simulink subsystem "transrapid_prebouclage"  (R2023a)
settings: Solver=VariableStepAuto  StartTime=0.0  StopTime=10.0  RelTol=1e-3
undefined symbols (not defined in the file): i0, k1, k2, kd, Ki, kp, Kz, Te, z0
libraries: dspsrcs4 x1
settings Model: Creator=leolebuhotel  LastModifiedBy=leolebuhotel

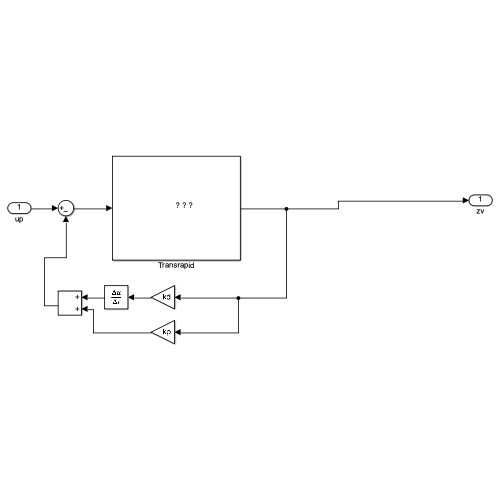
[thumbnail: Simulink's stored preview of the top-level diagram]
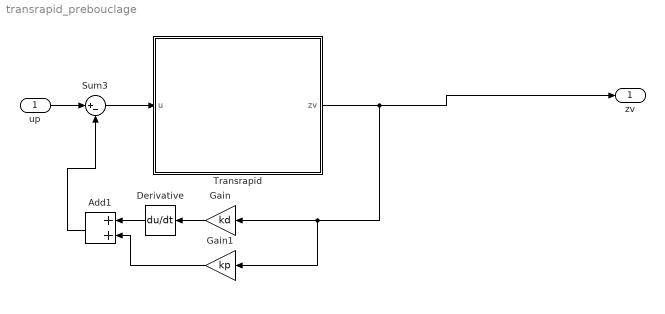
== system transrapid_prebouclage ==
  up : Inport
  Add1 : Sum
  Derivative : Derivative
  Gain : Gain  Gain=kd
  Gain1 : Gain  Gain=kp
  Sum3 : Sum  Inputs=|+-
  Transrapid : Subsystem
      mask Display:
      | image('Transrapid.jpg');
      | color('yellow')
      | port_label('output', 1, 'z');
      | port_label('input', 1, 'commande u');
  zv : Outport
  wires:
  Gain1/1 -> Add1/2
  Derivative/1 -> Add1/1
  up/1 -> Sum3/1
  Add1/1 -> Sum3/2
  Sum3/1 -> Transrapid/1(u)
  Transrapid/1(zv) -> zv/1, Gain1/1, Gain/1
  Gain/1 -> Derivative/1

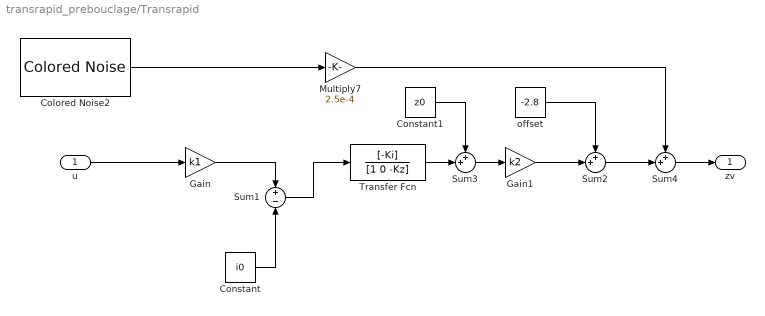
== system transrapid_prebouclage/Transrapid ==
  u : Inport
  Colored Noise2 : dspsrcs4/Colored Noise  Color=white  InverseFrequencyPower=1  BoundedOutput=off  NumChannels=1  OutputDataType=double  SamplesPerFrame=1  SampleTime=Te  RandomStream=mt19937ar with seed  Seed=67  SimulateUsing=Interpreted execution
  Constant : Constant  Value=i0
  Constant1 : Constant  Value=z0
  Gain : Gain  Gain=k1
  Gain1 : Gain  Gain=k2
  Multiply7 : Gain  Gain=2.5e-4
  Sum1 : Sum  Inputs=+-
  Sum2 : Sum  Inputs=++|
  Sum3 : Sum  Inputs=++|
  Sum4 : Sum  Inputs=++|
  Transfer Fcn : TransferFcn  Numerator=[-Ki]  Denominator=[1 0 -Kz]
  offset : Constant  Value=-2.8
  zv : Outport
  wires:
  Sum3/1 -> Gain1/1
  Transfer Fcn/1 -> Sum3/2
  Gain/1 -> Sum1/1
  Constant/1 -> Sum1/2
  Sum1/1 -> Transfer Fcn/1
  Constant1/1 -> Sum3/1
  Gain1/1 -> Sum2/2
  offset/1 -> Sum2/1
  Sum2/1 -> Sum4/2
  Sum4/1 -> zv/1
  Multiply7/1 -> Sum4/1
  Colored Noise2/1 -> Multiply7/1
  u/1 -> Gain/1
